simulink library "CommercialVehicleLibrary2G"  (R2021a)
settings: Solver=VariableStepAuto  StartTime=0.0  StopTime=10.0  RelTol=1e-3
values from neighbouring files (symbols this model uses):
  brake_input = [0   tmax ... (first row only)    [init_vehicle.m]    (also in run_Circle.m = [0  tmax; run_Coastdown.m = [0  2  tmax; run_DoubleLaneChangeDriver.m = [0   2  tmax; run_MaxAcc.m = [0  2  tmax)
  pose_t0 = [0 0 0 0]    [init_vehicle.m]    (also in run_Circle.m; run_Coastdown.m; run_DoubleLaneChangeDriver.m; run_MaxAcc.m)
  rdfname = 'TNO_FlatRoad.rdf'    [run_Circle.m]    (also in run_Coastdown.m; run_DoubleLaneChangeDriver.m; run_MaxAcc.m; run_Rollover.m)
  rdfname_inner = 'TNO_FlatRoad.rdf'    [run_Circle.m]    (also in run_Coastdown.m; run_DoubleLaneChangeDriver.m; run_MaxAcc.m; run_Rollover.m)
  steer_input = [0  tmax ... (first row only)    [init_vehicle.m]    (also in run_Circle.m = [0  2   10     13       tmax; run_Coastdown.m = [0 tmax; run_DoubleLaneChangeDriver.m = [0 tmax; run_MaxAcc.m = [0 tmax)
  throttle_input = [0         tmax ... (first row only)    [init_vehicle.m]    (also in run_Circle.m; run_Coastdown.m = [0        10         10.0001 tmax; run_DoubleLaneChangeDriver.m = [0        tmax; run_MaxAcc.m = [0        tmax)
  Vx = 0    [init_vehicle.m]    (also in run_Circle.m = Vx_kmh/3.6; run_Coastdown.m = Vx_kmh/3.6; run_DoubleLaneChangeDriver.m = Vx_kmh/3.6; run_MaxAcc.m)
  Vx_input = [0  tmax ... (first row only)    [init_vehicle.m]    (also in run_Circle.m; run_Coastdown.m = [0 tmax; run_DoubleLaneChangeDriver.m = [0 tmax; run_MaxAcc.m = [0 tmax)
undefined symbols (not defined in the file or in its folder): Drive, Floor, Fzstat, Fzstat1, Fzstat3, l, l_load1, l_load2, lbar, mass_load1, mass_load2, psi_semitrailer, rho, rim_Ixx, rim_Iyy, rim_mass, Steer, steer_path, tpfname, X, x_torsion, xcg, xcg1, xcg2, xcg_front, xcg_rear, xdrive1, xload1, xload2, xpos1, xref, xrev1, Xt0, Y, Yt0, Z
libraries: sm_lib x291, $bdroot x157, nesl_utility x143, vrlib x1
(part 5 of 12)

== system CommercialVehicleLibrary2G/Assemblies/Trailer load rear ==
  note: Measurements
  Bus Creator1 : BusCreator  Inputs=3
  Fcn1 : Fcn  Expr=u(2)
  Fcn2 : Fcn  Expr=u(2)
  "Load " : sm_lib/Body Elements/Brick Solid  GraphicAmbientColor=[0.15 0.15 0.15 1.0]  BasedOnType=Density  BrickDimensions=[l_load2 w h]  BrickDimensionUnits=m  CenterOfMass=[0 0 0]  CenterOfMassUnits=m  GraphicDiffuseColor=[1.0 1.0 0.2]  Density=1000  DensityUnits=kg/m^3  DoExposeReferenceFrame=on  GraphicEmissiveColor=[0.0 0.0 0.0 1.0]  ExportEntireGeometry=off  SerializedFrames=<Frames/>  MarkerShape=Sphere  MarkerSize=10  GraphicType=FromGeometry  InertiaType=Custom  Mass=mass_load  MassUnits=kg  MomentsOfInertia=[Ixx Iyy Izz]  MomentsOfInertiaUnits=kg*m^2  GraphicOpacity=0.5  ProductsOfInertia=[0 0 0]  ProductsOfInertiaUnits=kg*m^2  GraphicShininess=75  GraphicSpecularColor=[0.5 0.5 0.5 1.0]  GraphicVisPropType=SimpleVisualProperties
  Mux : Mux  Inputs=3
  Mux1 : Mux  Inputs=3
  Mux2 : Mux  Inputs=3
  PS-Simulink Converter : nesl_utility/PS-Simulink Converter  PhysicalDomain=network_engine_domain  SubClassName=ps_output  LeftPortType=input  RightPortType=output  PseudoPeriodic=off  Frequencies=[]  Unit=inherit  AffineConversion=off
      settings: SourceProductBaseCode=PW,SS
  PS-Simulink Converter{1..6} (6 alike) : nesl_utility/PS-Simulink Converter  PhysicalDomain=network_engine_domain  SubClassName=ps_output  LeftPortType=input  RightPortType=output  PseudoPeriodic=off  Frequencies=[]  Unit=m/s^2  AffineConversion=off
      settings: SourceProductBaseCode=PW,SS
  PS-Simulink Converter7 : nesl_utility/PS-Simulink Converter  PhysicalDomain=network_engine_domain  SubClassName=ps_output  LeftPortType=input  RightPortType=output  PseudoPeriodic=off  Frequencies=[]  Unit=inherit  AffineConversion=off
      settings: SourceProductBaseCode=PW,SS
  PS-Simulink Converter8 : nesl_utility/PS-Simulink Converter  PhysicalDomain=network_engine_domain  SubClassName=ps_output  LeftPortType=input  RightPortType=output  PseudoPeriodic=off  Frequencies=[]  Unit=inherit  AffineConversion=off
      settings: SourceProductBaseCode=PW,SS
  Transform Sensor : sm_lib/Frames and Transforms/Transform Sensor  MeasurementFrame=World  SenseAngle=off  SenseAxis=off  SenseAngle1=off  SenseAngle2=off  SenseAngle3=off  SenseQ=off  SenseR=off  SenseOmegaX=off  SenseOmegaY=off  SenseOmegaZ=off  SenseOmega1=off  SenseOmega2=off  SenseOmega3=off  SenseQDot=off  SenseRDot=off  SenseAlphaX=off  SenseAlphaY=off  SenseAlphaZ=off  SenseAlpha1=off  SenseAlpha2=off  SenseAlpha3=off  SenseQDDot=off  SenseRDDot=off  SenseX=on  SenseY=on  SenseZ=on  SenseRad=off  SenseAzim=off  SenseDist=off  SenseInc=off  SenseXDot=off  SenseYDot=off  SenseZDot=off  SenseRadDot=off  SenseAzimDot=off  SenseDistDot=off  SenseIncDot=off  SenseXDDot=off  SenseYDDot=off  SenseZDDot=off  SenseRadDDot=off  SenseAzimDDot=off  SenseDistDDot=off  SenseIncDDot=off
  Transform Sensor1 : sm_lib/Frames and Transforms/Transform Sensor  MeasurementFrame=NonRotatingFollower  SenseAngle=off  SenseAxis=off  SenseAngle1=off  SenseAngle2=off  SenseAngle3=off  SenseQ=off  SenseR=off  SenseOmegaX=off  SenseOmegaY=off  SenseOmegaZ=off  SenseOmega1=off  SenseOmega2=off  SenseOmega3=off  SenseQDot=off  SenseRDot=off  SenseAlphaX=off  SenseAlphaY=off  SenseAlphaZ=off  SenseAlpha1=off  SenseAlpha2=off  SenseAlpha3=off  SenseQDDot=off  SenseRDDot=off  SenseX=off  SenseY=off  SenseZ=off  SenseRad=off  SenseAzim=off  SenseDist=off  SenseInc=off  SenseXDot=off  SenseYDot=off  SenseZDot=off  SenseRadDot=off  SenseAzimDot=off  SenseDistDot=off  SenseIncDot=off  SenseXDDot=on  SenseYDDot=on  SenseZDDot=on  SenseRadDDot=off  SenseAzimDDot=off  SenseDistDDot=off  SenseIncDDot=off
  Transform Sensor2 : sm_lib/Frames and Transforms/Transform Sensor  MeasurementFrame=NonRotatingFollower  SenseAngle=off  SenseAxis=off  SenseAngle1=off  SenseAngle2=off  SenseAngle3=off  SenseQ=off  SenseR=off  SenseOmegaX=off  SenseOmegaY=off  SenseOmegaZ=off  SenseOmega1=off  SenseOmega2=off  SenseOmega3=off  SenseQDot=off  SenseRDot=off  SenseAlphaX=off  SenseAlphaY=off  SenseAlphaZ=off  SenseAlpha1=off  SenseAlpha2=off  SenseAlpha3=off  SenseQDDot=off  SenseRDDot=off  SenseX=off  SenseY=off  SenseZ=off  SenseRad=off  SenseAzim=off  SenseDist=off  SenseInc=off  SenseXDot=off  SenseYDot=off  SenseZDot=off  SenseRadDot=off  SenseAzimDot=off  SenseDistDot=off  SenseIncDot=off  SenseXDDot=on  SenseYDDot=on  SenseZDDot=on  SenseRadDDot=off  SenseAzimDDot=off  SenseDistDDot=off  SenseIncDDot=off
  Weld Joint : sm_lib/Joints/Weld Joint  JointMode=Normal  SenseConstraintForce=off  SenseConstraintForceX=off  SenseConstraintForceY=off  SenseConstraintForceZ=off  SenseConstraintTorque=off  SenseConstraintTorqueX=off  SenseConstraintTorqueY=off  SenseConstraintTorqueZ=off  SenseTotalForce=off  SenseTotalForceX=off  SenseTotalForceY=off  SenseTotalForceZ=off  SenseTotalTorque=off  SenseTotalTorqueX=off  SenseTotalTorqueY=off  SenseTotalTorqueZ=off  CompositeWrenchDir=FollowerOnBase  CompositeWrenchFrame=BaseFrame
  World Frame : sm_lib/Frames and Transforms/World Frame
  World Frame1 : sm_lib/Frames and Transforms/World Frame
  World Frame2 : sm_lib/Frames and Transforms/World Frame
  load_corner_pos : sm_lib/Frames and Transforms/Rigid Transform  TranslationMethod=Cartesian  TranslationStandardOffset=0  TranslationLengthUnit=m  TranslationStandardAxis=+Z  TranslationCartesianOffset=[(-0.5*l_load) 0 0]  TranslationROffset=0  TranslationROffsetUnits=m  TranslationZOffset=0  TranslationZOffsetUnits=m  TranslationThetaOffset=0  TranslationThetaOffsetUnits=deg  RotationMethod=None  RotationAngleUnits=deg  RotationStandardAxis=+Z  RotationAngle=0.0  RotationArbitraryAxis=[0 0 1]  FollAlignAxisA=+X  BaseAlignAxisA=+Y  FollAlignAxisB=+Y  BaseAlignAxisB=+Z  RotationSequenceAxes=FollowerAxes  RotationSequence=XYX  RotationSequenceAngles=[0 0 0]  RotationSequenceAnglesUnits=deg  RotationMatrix=[1 0 0; 0 1 0; 0 0 1]
  pos_load : sm_lib/Frames and Transforms/Rigid Transform  TranslationMethod=Cartesian  TranslationStandardOffset=0  TranslationLengthUnit=m  TranslationStandardAxis=+Z  TranslationCartesianOffset=[-xcg2+xload 0 zcg+0.1]  TranslationROffset=0  TranslationROffsetUnits=m  TranslationZOffset=0  TranslationZOffsetUnits=m  TranslationThetaOffset=0  TranslationThetaOffsetUnits=deg  RotationMethod=None  RotationAngleUnits=deg  RotationStandardAxis=+Z  RotationAngle=0.0  RotationArbitraryAxis=[0 0 1]  FollAlignAxisA=+X  BaseAlignAxisA=+Y  FollAlignAxisB=+Y  BaseAlignAxisB=+Z  RotationSequenceAxes=FollowerAxes  RotationSequence=XYX  RotationSequenceAngles=[0 0 0]  RotationSequenceAnglesUnits=deg  RotationMatrix=[1 0 0; 0 1 0; 0 0 1]
  Chassis : PMIOPort  Side=Left
  Out1 : Outport
  wires:
  PS-Simulink Converter7/1 -> Mux/2
  PS-Simulink Converter/1 -> Mux/1
  PS-Simulink Converter8/1 -> Mux/3
  PS-Simulink Converter3/1 -> Mux1/1
  Mux1/1 -> Fcn2/1
  Mux/1 -> [Load_pos]
  PS-Simulink Converter5/1 -> Mux1/3
  Fcn2/1 -> [Load_acc_center]
  PS-Simulink Converter4/1 -> Mux1/2
  [Load_acc_center] -> Bus Creator1/2  "acc_center"
  Bus Creator1/1 -> Out1/1
  [Load_pos] -> Bus Creator1/1  "pos"
  PS-Simulink Converter2/1 -> Mux2/2
  PS-Simulink Converter1/1 -> Mux2/1
  PS-Simulink Converter6/1 -> Mux2/3
  Mux2/1 -> Fcn1/1
  Fcn1/1 -> [Load_acc_corner]
  [Load_acc_corner] -> Bus Creator1/3  "acc_corner"
  connections:
  "Load "/RConn1 -- Transform Sensor2/RConn1 -- Transform Sensor/RConn1 -- load_corner_pos/LConn1 -- pos_load/RConn1
  PS-Simulink Converter8/LConn1 -- Transform Sensor/RConn4
  PS-Simulink Converter7/LConn1 -- Transform Sensor/RConn3
  PS-Simulink Converter4/LConn1 -- Transform Sensor2/RConn3
  World Frame/RConn1 -- Transform Sensor/LConn1
  PS-Simulink Converter3/LConn1 -- Transform Sensor2/RConn2
  PS-Simulink Converter5/LConn1 -- Transform Sensor2/RConn4
  PS-Simulink Converter/LConn1 -- Transform Sensor/RConn2
  World Frame2/RConn1 -- Transform Sensor2/LConn1
  pos_load/LConn1 -- Weld Joint/RConn1
  Weld Joint/LConn1 -- Chassis/RConn1
  PS-Simulink Converter6/LConn1 -- Transform Sensor1/RConn4
  World Frame1/RConn1 -- Transform Sensor1/LConn1
  Transform Sensor1/RConn1 -- load_corner_pos/RConn1
  PS-Simulink Converter1/LConn1 -- Transform Sensor1/RConn2
  PS-Simulink Converter2/LConn1 -- Transform Sensor1/RConn3

== system CommercialVehicleLibrary2G/Assemblies/Truck load ==
  note: Measurements
  Bus Creator1 : BusCreator  Inputs=3
  Fcn1 : Fcn  Expr=u(2)
  Fcn2 : Fcn  Expr=u(2)
  "Load " : sm_lib/Body Elements/Brick Solid  GraphicAmbientColor=[0.15 0.15 0.15 1.0]  BasedOnType=Density  BrickDimensions=[l_load w h]  BrickDimensionUnits=m  CenterOfMass=[0 0 0]  CenterOfMassUnits=m  GraphicDiffuseColor=[1.0 0.4 0.4]  Density=1000  DensityUnits=kg/m^3  DoExposeReferenceFrame=on  GraphicEmissiveColor=[0.0 0.0 0.0 1.0]  ExportEntireGeometry=off  SerializedFrames=<Frames/>  MarkerShape=Sphere  MarkerSize=10  GraphicType=FromGeometry  InertiaType=Custom  Mass=mass_load  MassUnits=kg  MomentsOfInertia=[Ixx Iyy Izz]  MomentsOfInertiaUnits=kg*m^2  GraphicOpacity=0.5  ProductsOfInertia=[0 0 0]  ProductsOfInertiaUnits=kg*m^2  GraphicShininess=75  GraphicSpecularColor=[0.5 0.5 0.5 1.0]  GraphicVisPropType=SimpleVisualProperties
  Mux : Mux  Inputs=3
  Mux1 : Mux  Inputs=3
  Mux2 : Mux  Inputs=3
  PS-Simulink Converter : nesl_utility/PS-Simulink Converter  PhysicalDomain=network_engine_domain  SubClassName=ps_output  LeftPortType=input  RightPortType=output  PseudoPeriodic=off  Frequencies=[]  Unit=inherit  AffineConversion=off
      settings: SourceProductBaseCode=PW,SS
  PS-Simulink Converter{1..6} (6 alike) : nesl_utility/PS-Simulink Converter  PhysicalDomain=network_engine_domain  SubClassName=ps_output  LeftPortType=input  RightPortType=output  PseudoPeriodic=off  Frequencies=[]  Unit=m/s^2  AffineConversion=off
      settings: SourceProductBaseCode=PW,SS
  PS-Simulink Converter7 : nesl_utility/PS-Simulink Converter  PhysicalDomain=network_engine_domain  SubClassName=ps_output  LeftPortType=input  RightPortType=output  PseudoPeriodic=off  Frequencies=[]  Unit=inherit  AffineConversion=off
      settings: SourceProductBaseCode=PW,SS
  PS-Simulink Converter8 : nesl_utility/PS-Simulink Converter  PhysicalDomain=network_engine_domain  SubClassName=ps_output  LeftPortType=input  RightPortType=output  PseudoPeriodic=off  Frequencies=[]  Unit=inherit  AffineConversion=off
      settings: SourceProductBaseCode=PW,SS
  Transform Sensor : sm_lib/Frames and Transforms/Transform Sensor  MeasurementFrame=World  SenseAngle=off  SenseAxis=off  SenseAngle1=off  SenseAngle2=off  SenseAngle3=off  SenseQ=off  SenseR=off  SenseOmegaX=off  SenseOmegaY=off  SenseOmegaZ=off  SenseOmega1=off  SenseOmega2=off  SenseOmega3=off  SenseQDot=off  SenseRDot=off  SenseAlphaX=off  SenseAlphaY=off  SenseAlphaZ=off  SenseAlpha1=off  SenseAlpha2=off  SenseAlpha3=off  SenseQDDot=off  SenseRDDot=off  SenseX=on  SenseY=on  SenseZ=on  SenseRad=off  SenseAzim=off  SenseDist=off  SenseInc=off  SenseXDot=off  SenseYDot=off  SenseZDot=off  SenseRadDot=off  SenseAzimDot=off  SenseDistDot=off  SenseIncDot=off  SenseXDDot=off  SenseYDDot=off  SenseZDDot=off  SenseRadDDot=off  SenseAzimDDot=off  SenseDistDDot=off  SenseIncDDot=off
  Transform Sensor1 : sm_lib/Frames and Transforms/Transform Sensor  MeasurementFrame=NonRotatingFollower  SenseAngle=off  SenseAxis=off  SenseAngle1=off  SenseAngle2=off  SenseAngle3=off  SenseQ=off  SenseR=off  SenseOmegaX=off  SenseOmegaY=off  SenseOmegaZ=off  SenseOmega1=off  SenseOmega2=off  SenseOmega3=off  SenseQDot=off  SenseRDot=off  SenseAlphaX=off  SenseAlphaY=off  SenseAlphaZ=off  SenseAlpha1=off  SenseAlpha2=off  SenseAlpha3=off  SenseQDDot=off  SenseRDDot=off  SenseX=off  SenseY=off  SenseZ=off  SenseRad=off  SenseAzim=off  SenseDist=off  SenseInc=off  SenseXDot=off  SenseYDot=off  SenseZDot=off  SenseRadDot=off  SenseAzimDot=off  SenseDistDot=off  SenseIncDot=off  SenseXDDot=on  SenseYDDot=on  SenseZDDot=on  SenseRadDDot=off  SenseAzimDDot=off  SenseDistDDot=off  SenseIncDDot=off
  Transform Sensor2 : sm_lib/Frames and Transforms/Transform Sensor  MeasurementFrame=NonRotatingFollower  SenseAngle=off  SenseAxis=off  SenseAngle1=off  SenseAngle2=off  SenseAngle3=off  SenseQ=off  SenseR=off  SenseOmegaX=off  SenseOmegaY=off  SenseOmegaZ=off  SenseOmega1=off  SenseOmega2=off  SenseOmega3=off  SenseQDot=off  SenseRDot=off  SenseAlphaX=off  SenseAlphaY=off  SenseAlphaZ=off  SenseAlpha1=off  SenseAlpha2=off  SenseAlpha3=off  SenseQDDot=off  SenseRDDot=off  SenseX=off  SenseY=off  SenseZ=off  SenseRad=off  SenseAzim=off  SenseDist=off  SenseInc=off  SenseXDot=off  SenseYDot=off  SenseZDot=off  SenseRadDot=off  SenseAzimDot=off  SenseDistDot=off  SenseIncDot=off  SenseXDDot=on  SenseYDDot=on  SenseZDDot=on  SenseRadDDot=off  SenseAzimDDot=off  SenseDistDDot=off  SenseIncDDot=off
  Weld Joint : sm_lib/Joints/Weld Joint  JointMode=Normal  SenseConstraintForce=off  SenseConstraintForceX=off  SenseConstraintForceY=off  SenseConstraintForceZ=off  SenseConstraintTorque=off  SenseConstraintTorqueX=off  SenseConstraintTorqueY=off  SenseConstraintTorqueZ=off  SenseTotalForce=off  SenseTotalForceX=off  SenseTotalForceY=off  SenseTotalForceZ=off  SenseTotalTorque=off  SenseTotalTorqueX=off  SenseTotalTorqueY=off  SenseTotalTorqueZ=off  CompositeWrenchDir=FollowerOnBase  CompositeWrenchFrame=BaseFrame
  World Frame : sm_lib/Frames and Transforms/World Frame
  World Frame1 : sm_lib/Frames and Transforms/World Frame
  World Frame2 : sm_lib/Frames and Transforms/World Frame
  load_corner_pos : sm_lib/Frames and Transforms/Rigid Transform  TranslationMethod=Cartesian  TranslationStandardOffset=0  TranslationLengthUnit=m  TranslationStandardAxis=+Z  TranslationCartesianOffset=[(-0.5*l_load) 0 0]  TranslationROffset=0  TranslationROffsetUnits=m  TranslationZOffset=0  TranslationZOffsetUnits=m  TranslationThetaOffset=0  TranslationThetaOffsetUnits=deg  RotationMethod=None  RotationAngleUnits=deg  RotationStandardAxis=+Z  RotationAngle=0.0  RotationArbitraryAxis=[0 0 1]  FollAlignAxisA=+X  BaseAlignAxisA=+Y  FollAlignAxisB=+Y  BaseAlignAxisB=+Z  RotationSequenceAxes=FollowerAxes  RotationSequence=XYX  RotationSequenceAngles=[0 0 0]  RotationSequenceAnglesUnits=deg  RotationMatrix=[1 0 0; 0 1 0; 0 0 1]
  pos_load : sm_lib/Frames and Transforms/Rigid Transform  TranslationMethod=Cartesian  TranslationStandardOffset=0  TranslationLengthUnit=m  TranslationStandardAxis=+Z  TranslationCartesianOffset=[-xcg_rear+xload 0 +zload+zcg-0.9]  TranslationROffset=0  TranslationROffsetUnits=m  TranslationZOffset=0  TranslationZOffsetUnits=m  TranslationThetaOffset=0  TranslationThetaOffsetUnits=deg  RotationMethod=None  RotationAngleUnits=deg  RotationStandardAxis=+Z  RotationAngle=0.0  RotationArbitraryAxis=[0 0 1]  FollAlignAxisA=+X  BaseAlignAxisA=+Y  FollAlignAxisB=+Y  BaseAlignAxisB=+Z  RotationSequenceAxes=FollowerAxes  RotationSequence=XYX  RotationSequenceAngles=[0 0 0]  RotationSequenceAnglesUnits=deg  RotationMatrix=[1 0 0; 0 1 0; 0 0 1]
  Chassis : PMIOPort  Side=Left
  Out1 : Outport
  wires:
  [Load_acc_corner] -> Bus Creator1/3  "acc_corner"
  Fcn1/1 -> [Load_acc_corner]
  Mux2/1 -> Fcn1/1
  PS-Simulink Converter6/1 -> Mux2/3
  PS-Simulink Converter1/1 -> Mux2/1
  PS-Simulink Converter2/1 -> Mux2/2
  [Load_pos] -> Bus Creator1/1  "pos"
  Bus Creator1/1 -> Out1/1
  [Load_acc_center] -> Bus Creator1/2  "acc_center"
  PS-Simulink Converter4/1 -> Mux1/2
  Fcn2/1 -> [Load_acc_center]
  PS-Simulink Converter5/1 -> Mux1/3
  Mux/1 -> [Load_pos]
  Mux1/1 -> Fcn2/1
  PS-Simulink Converter3/1 -> Mux1/1
  PS-Simulink Converter8/1 -> Mux/3
  PS-Simulink Converter/1 -> Mux/1
  PS-Simulink Converter7/1 -> Mux/2
  connections:
  PS-Simulink Converter2/LConn1 -- Transform Sensor1/RConn3
  PS-Simulink Converter1/LConn1 -- Transform Sensor1/RConn2
  Transform Sensor1/RConn1 -- load_corner_pos/RConn1
  World Frame1/RConn1 -- Transform Sensor1/LConn1
  PS-Simulink Converter6/LConn1 -- Transform Sensor1/RConn4
  Weld Joint/LConn1 -- Chassis/RConn1
  pos_load/LConn1 -- Weld Joint/RConn1
  World Frame2/RConn1 -- Transform Sensor2/LConn1
  PS-Simulink Converter/LConn1 -- Transform Sensor/RConn2
  PS-Simulink Converter5/LConn1 -- Transform Sensor2/RConn4
  PS-Simulink Converter3/LConn1 -- Transform Sensor2/RConn2
  World Frame/RConn1 -- Transform Sensor/LConn1
  PS-Simulink Converter4/LConn1 -- Transform Sensor2/RConn3
  PS-Simulink Converter7/LConn1 -- Transform Sensor/RConn3
  PS-Simulink Converter8/LConn1 -- Transform Sensor/RConn4
  pos_load/RConn1 -- load_corner_pos/LConn1 -- Transform Sensor/RConn1 -- Transform Sensor2/RConn1 -- "Load "/RConn1

== system CommercialVehicleLibrary2G/Combinations/LZV_A ==
  Bus Selector : BusSelector  OutputSignals=chassis.Vx,steeraxle.pos,driveaxle.pos
  Clock : Clock
  "Drawbar Trailer - 2 axle " : $bdroot/Trailers/Drawbar Trailer - 2 axle   xref=-15.06+1  l_chassis=7.82  lbar=2.0  mass_empty=3900  mass_load=13600  rho=350  Fzstat=8500*9.81
  Driver : $bdroot/Assemblies/Driver  SystemSampleTime=-1  VariantActivationTime=update diagram  Latency=0  AutoFrameSizeCalculation=off
  Semitrailer : $bdroot/Trailers/Semitrailer  xref=-3.06  xaxle2=8.475  lchassis=13.6  x5th=1.6  mass_empty=6000  mass_load=27000  rho=350  Fzstat=7200*9.81  lbdouble=0  psi_semitrailer=pose_t0(4)
  To Workspace : ToWorkspace  VariableName=p_time  SampleTime=-1
  To Workspace21 : ToWorkspace  VariableName=p_inputs_delta  SampleTime=-1
  To Workspace22 : ToWorkspace  VariableName=p_inputs_throttle  SampleTime=-1
  To Workspace23 : ToWorkspace  VariableName=p_inputs_brake  SampleTime=-1
  To_workspace_drawbar_trailer_2axle : $bdroot/Utilities/To_workspace_drawbar_trailer_2axle  SystemSampleTime=-1  VariantActivationTime=update diagram  Latency=0  AutoFrameSizeCalculation=off
  To_workspace_semitrailer : $bdroot/Utilities/To_workspace_semitrailer  SystemSampleTime=-1  VariantActivationTime=update diagram  Latency=0  AutoFrameSizeCalculation=off
  To_workspace_tractor : $bdroot/Utilities/To_workspace_tractor  SystemSampleTime=-1  VariantActivationTime=update diagram  Latency=0  AutoFrameSizeCalculation=off
  Tractor : $bdroot/Vehicles/Tractor  xref=0  xrear=-3.80  Fzstat1=7500*9.81  Fzstat2=11500*9.81  Xt0=pose_t0(1)  Yt0=pose_t0(2)  Psit0=pose_t0(3)
  wires:
  Driver/3 -> Tractor/3, To Workspace23/1
  Driver/2 -> Tractor/2, To Workspace22/1
  Clock/1 -> Driver/1, To Workspace/1
  Driver/1 -> Tractor/1, To Workspace21/1
  Tractor/1 -> To_workspace_tractor/1, Bus Selector/1
  Bus Selector/1 -> Driver/2  "<Vx>"
  Bus Selector/2 -> Driver/3  "<pos>"
  Bus Selector/3 -> Driver/4  "<pos>"
  Tractor/2 -> Semitrailer/1, "Drawbar Trailer - 2 axle "/1
  "Drawbar Trailer - 2 axle "/1 -> To_workspace_drawbar_trailer_2axle/1
  Semitrailer/1 -> To_workspace_semitrailer/1
  connections:
  Semitrailer/LConn1 -- Tractor/RConn1
  Semitrailer/RConn1 -- "Drawbar Trailer - 2 axle "/LConn1

== system CommercialVehicleLibrary2G/Combinations/LZV_B ==
  Bus Selector : BusSelector  OutputSignals=chassis.Vx,steeraxle.pos,driveaxle.pos
  Clock : Clock
  Driver : $bdroot/Assemblies/Driver  SystemSampleTime=-1  VariantActivationTime=update diagram  Latency=0  AutoFrameSizeCalculation=off
  Semitrailer : $bdroot/Trailers/Semitrailer  xref=-3.06  xaxle2=8.475  lchassis=12.0  x5th=1.6  mass_empty=5000  mass_load=14500  rho=350  Fzstat=6400*9.81  lbdouble=4.18  psi_semitrailer=pose_t0(4)
  Semitrailer1 : $bdroot/Trailers/Semitrailer  xref=-11.85  xaxle2=8.475  lchassis=13.6  x5th=1.6  mass_empty=6000  mass_load=25000  rho=350  Fzstat=6600*9.81  lbdouble=0  psi_semitrailer=pose_t0(4)
  To Workspace : ToWorkspace  VariableName=p_time  SampleTime=-1
  To Workspace21 : ToWorkspace  VariableName=p_inputs_delta  SampleTime=-1
  To Workspace22 : ToWorkspace  VariableName=p_inputs_throttle  SampleTime=-1
  To Workspace23 : ToWorkspace  VariableName=p_inputs_brake  SampleTime=-1
  To_workspace_semitrailer1 : Subsystem
  To_workspace_semitrailer2 : Subsystem
  To_workspace_tractor : $bdroot/Utilities/To_workspace_tractor  SystemSampleTime=-1  VariantActivationTime=update diagram  Latency=0  AutoFrameSizeCalculation=off
  Tractor : $bdroot/Vehicles/Tractor  xref=0  xrear=-3.80  Fzstat1=7500*9.81  Fzstat2=11500*9.81  Xt0=pose_t0(1)  Yt0=pose_t0(2)  Psit0=pose_t0(3)
  wires:
  Driver/3 -> Tractor/3, To Workspace23/1
  Driver/2 -> Tractor/2, To Workspace22/1
  Clock/1 -> Driver/1, To Workspace/1
  Driver/1 -> Tractor/1, To Workspace21/1
  Tractor/1 -> To_workspace_tractor/1, Bus Selector/1
  Bus Selector/1 -> Driver/2  "<Vx>"
  Bus Selector/2 -> Driver/3  "<pos>"
  Bus Selector/3 -> Driver/4  "<pos>"
  Semitrailer1/1 -> To_workspace_semitrailer2/1(In1)
  Tractor/2 -> Semitrailer1/1, Semitrailer/1
  Semitrailer/1 -> To_workspace_semitrailer1/1(In1)
  connections:
  Semitrailer/LConn1 -- Tractor/RConn1
  Semitrailer1/LConn1 -- Semitrailer/RConn1

== system CommercialVehicleLibrary2G/Combinations/LZV_C ==
  Bus Selector : BusSelector  OutputSignals=chassis.Vx,steeraxle1.pos,driveaxle2.pos
  Clock : Clock
  Driver : $bdroot/Assemblies/Driver  SystemSampleTime=-1  VariantActivationTime=update diagram  Latency=0  AutoFrameSizeCalculation=off
  Rigid Truck - 4 axles : $bdroot/Vehicles/Rigid Truck - 4 axles  xref=0  xaxle=5.1  l_chassis=12  l_load=9.6  mass_load=19000  rho=350  Fzstat1=7500*9.81  Fzstat2=7500*9.81  Fzstat3=8500*9.81  Fzstat4=8500*9.81  conf=Steer-Steer-Drive-Drive  Xt0=pose_t0(1)  Yt0=pose_t0(2)  Psit0=pose_t0(3)
  To Workspace : ToWorkspace  VariableName=p_time  SampleTime=-1
  To Workspace21 : ToWorkspace  VariableName=p_inputs_delta  SampleTime=-1
  To Workspace22 : ToWorkspace  VariableName=p_inputs_throttle  SampleTime=-1
  To Workspace23 : ToWorkspace  VariableName=p_inputs_brake  SampleTime=-1
  To_workspace_trailer_3axle : $bdroot/Utilities/To_workspace_trailer_3axle  SystemSampleTime=-1  VariantActivationTime=update diagram  Latency=0  AutoFrameSizeCalculation=off
  To_workspace_truck_4axle1 : $bdroot/Utilities/To_workspace_truck_4axle  SystemSampleTime=-1  VariantActivationTime=update diagram  Latency=0  AutoFrameSizeCalculation=off
  "Trailer - 3 axle " : $bdroot/Trailers/Trailer - 3 axle   xref=-10.0  xtrailer=5  l_chassis=10  lturn=1.2  lbar=2.7  mass_empty=6000  mass_load=22000  rho=350  Fzstat=9333*9.81
  wires:
  Driver/3 -> Rigid Truck - 4 axles/3, To Workspace23/1
  Driver/2 -> Rigid Truck - 4 axles/2, To Workspace22/1
  Clock/1 -> Driver/1, To Workspace/1
  Driver/1 -> Rigid Truck - 4 axles/1, To Workspace21/1
  Rigid Truck - 4 axles/1 -> To_workspace_truck_4axle1/1, Bus Selector/1
  Bus Selector/1 -> Driver/2  "<Vx>"
  Bus Selector/2 -> Driver/3  "<pos>"
  Bus Selector/3 -> Driver/4  "<pos>"
  "Trailer - 3 axle "/1 -> To_workspace_trailer_3axle/1
  Rigid Truck - 4 axles/2 -> "Trailer - 3 axle "/1
  connections:
  "Trailer - 3 axle "/LConn1 -- Rigid Truck - 4 axles/RConn1

== system CommercialVehicleLibrary2G/Combinations/LZV_D ==
  Bus Selector : BusSelector  OutputSignals=chassis.Vx,steeraxle.pos,driveaxle2.pos
  Clock : Clock
  Dolly : $bdroot/Trailers/Dolly  xref=-8.35  lbar=3.50  Fzstat=6700*9.81
  Driver : $bdroot/Assemblies/Driver  SystemSampleTime=-1  VariantActivationTime=update diagram  Latency=0  AutoFrameSizeCalculation=off
  Rigid Truck - 3 axles : $bdroot/Vehicles/Rigid Truck - 3 axles  xref=0  xaxle=5.0  l_load=7.82  mass_load=15000  rho=350  Fzstat1=7500*9.81  Fzstat2=9250*9.81  Fzstat3=9250*9.81  Xt0=pose_t0(1)  Yt0=pose_t0(2)  Psit0=pose_t0(3)
  Semitrailer : $bdroot/Trailers/Semitrailer  xref=-11.85  xaxle2=8.475  lchassis=13.6  x5th=1.6  mass_empty=6000  mass_load=26200  rho=350  Fzstat=6800*9.81  lbdouble=0  psi_semitrailer=pose_t0(4)
  To Workspace : ToWorkspace  VariableName=p_time  SampleTime=-1
  To Workspace21 : ToWorkspace  VariableName=p_inputs_delta  SampleTime=-1
  To Workspace22 : ToWorkspace  VariableName=p_inputs_throttle  SampleTime=-1
  To Workspace23 : ToWorkspace  VariableName=p_inputs_brake  SampleTime=-1
  To_workspace_dolly : $bdroot/Utilities/To_workspace_dolly  SystemSampleTime=-1  VariantActivationTime=update diagram  Latency=0  AutoFrameSizeCalculation=off
  To_workspace_semitrailer : $bdroot/Utilities/To_workspace_semitrailer  SystemSampleTime=-1  VariantActivationTime=update diagram  Latency=0  AutoFrameSizeCalculation=off
  To_workspace_truck_3axle : $bdroot/Utilities/To_workspace_truck_3axle  SystemSampleTime=-1  VariantActivationTime=update diagram  Latency=0  AutoFrameSizeCalculation=off
  wires:
  Driver/3 -> Rigid Truck - 3 axles/3, To Workspace23/1
  Driver/2 -> Rigid Truck - 3 axles/2, To Workspace22/1
  Clock/1 -> Driver/1, To Workspace/1
  Driver/1 -> Rigid Truck - 3 axles/1, To Workspace21/1
  Rigid Truck - 3 axles/1 -> To_workspace_truck_3axle/1, Bus Selector/1
  Bus Selector/1 -> Driver/2  "<Vx>"
  Dolly/1 -> To_workspace_dolly/1
  Bus Selector/2 -> Driver/3  "<pos>"
  Bus Selector/3 -> Driver/4  "<pos>"
  Rigid Truck - 3 axles/2 -> Semitrailer/1, Dolly/1
  Semitrailer/1 -> To_workspace_semitrailer/1
  connections:
  Dolly/LConn1 -- Rigid Truck - 3 axles/RConn1
  Semitrailer/LConn1 -- Dolly/RConn1

== system CommercialVehicleLibrary2G/Combinations/LZV_E ==
  Bus Selector : BusSelector  OutputSignals=chassis.Vx,steeraxle.pos,driveaxle2.pos
  Clock : Clock
  "Drawbar Trailer - 2 axle 1 " : $bdroot/Trailers/Drawbar Trailer - 2 axle   xref=-7.82  l_chassis=6.5  lbar=2.0  mass_empty=4000  mass_load=13000  rho=350  Fzstat=8600*9.81
  Drawbar Trailer - 2 axle 2 : $bdroot/Trailers/Drawbar Trailer - 2 axle   xref=-15.32  l_chassis=6.5  lbar=2.0  mass_empty=4000  mass_load=13000  rho=350  Fzstat=8250*9.81
  Driver : $bdroot/Assemblies/Driver  SystemSampleTime=-1  VariantActivationTime=update diagram  Latency=0  AutoFrameSizeCalculation=off
  Rigid Truck - 3 axles : $bdroot/Vehicles/Rigid Truck - 3 axles  xref=0  xaxle=5.0  l_load=7.82  mass_load=15000  rho=350  Fzstat1=7400*9.81  Fzstat2=9450*9.81  Fzstat3=9450*9.81  Xt0=pose_t0(1)  Yt0=pose_t0(2)  Psit0=pose_t0(3)
  To Workspace : ToWorkspace  VariableName=p_time  SampleTime=-1
  To Workspace21 : ToWorkspace  VariableName=p_inputs_delta  SampleTime=-1
  To Workspace22 : ToWorkspace  VariableName=p_inputs_throttle  SampleTime=-1
  To Workspace23 : ToWorkspace  VariableName=p_inputs_brake  SampleTime=-1
  To_workspace_drawbar_trailer_2axle : $bdroot/Utilities/To_workspace_drawbar_trailer_2axle  SystemSampleTime=-1  VariantActivationTime=update diagram  Latency=0  AutoFrameSizeCalculation=off
  To_workspace_drawbar_trailer_2axle 2 : Subsystem
  To_workspace_truck_3axle : $bdroot/Utilities/To_workspace_truck_3axle  SystemSampleTime=-1  VariantActivationTime=update diagram  Latency=0  AutoFrameSizeCalculation=off
  wires:
  Driver/3 -> Rigid Truck - 3 axles/3, To Workspace23/1
  Driver/2 -> Rigid Truck - 3 axles/2, To Workspace22/1
  Clock/1 -> Driver/1, To Workspace/1
  Driver/1 -> Rigid Truck - 3 axles/1, To Workspace21/1
  Rigid Truck - 3 axles/1 -> To_workspace_truck_3axle/1, Bus Selector/1
  Bus Selector/1 -> Driver/2  "<Vx>"
  "Drawbar Trailer - 2 axle 1 "/1 -> To_workspace_drawbar_trailer_2axle/1
  Bus Selector/2 -> Driver/3  "<pos>"
  Bus Selector/3 -> Driver/4  "<pos>"
  Rigid Truck - 3 axles/2 -> Drawbar Trailer - 2 axle 2/1, "Drawbar Trailer - 2 axle 1 "/1
  Drawbar Trailer - 2 axle 2/1 -> To_workspace_drawbar_trailer_2axle 2/1(In1)
  connections:
  "Drawbar Trailer - 2 axle 1 "/LConn1 -- Rigid Truck - 3 axles/RConn1
  Drawbar Trailer - 2 axle 2/LConn1 -- "Drawbar Trailer - 2 axle 1 "/RConn1

== system CommercialVehicleLibrary2G/Combinations/LZV_F ==
  Bus Selector : BusSelector  OutputSignals=chassis.Vx,steeraxle1.pos,driveaxle2.pos
  Clock : Clock
  Driver : $bdroot/Assemblies/Driver  SystemSampleTime=-1  VariantActivationTime=update diagram  Latency=0  AutoFrameSizeCalculation=off
  Rigid Truck - 4 axles : $bdroot/Vehicles/Rigid Truck - 4 axles  xref=0  xaxle=5.25  l_chassis=10.1  l_load=5  mass_load=10000  rho=350  Fzstat1=7500*9.81  Fzstat2=7500*9.81  Fzstat3=10000*9.81  Fzstat4=10000*9.81  conf=Steer-Drive-Drive-Steer  Xt0=pose_t0(1)  Yt0=pose_t0(2)  Psit0=pose_t0(3)
  Semitrailer : $bdroot/Trailers/Semitrailer  xref=-8.4  xaxle2=8.475  lchassis=13.6  x5th=1.6  mass_empty=6000  mass_load=27000  rho=350  Fzstat=7000*9.81  lbdouble=0  psi_semitrailer=pose_t0(4)
  To Workspace : ToWorkspace  VariableName=p_time  SampleTime=-1
  To Workspace21 : ToWorkspace  VariableName=p_inputs_delta  SampleTime=-1
  To Workspace22 : ToWorkspace  VariableName=p_inputs_throttle  SampleTime=-1
  To Workspace23 : ToWorkspace  VariableName=p_inputs_brake  SampleTime=-1
  To_workspace_semitrailer : $bdroot/Utilities/To_workspace_semitrailer  SystemSampleTime=-1  VariantActivationTime=update diagram  Latency=0  AutoFrameSizeCalculation=off
  To_workspace_truck_4axle : $bdroot/Utilities/To_workspace_truck_4axle  SystemSampleTime=-1  VariantActivationTime=update diagram  Latency=0  AutoFrameSizeCalculation=off
  wires:
  Driver/3 -> Rigid Truck - 4 axles/3, To Workspace23/1
  Driver/2 -> Rigid Truck - 4 axles/2, To Workspace22/1
  Clock/1 -> Driver/1, To Workspace/1
  Driver/1 -> Rigid Truck - 4 axles/1, To Workspace21/1
  Rigid Truck - 4 axles/1 -> To_workspace_truck_4axle/1, Bus Selector/1
  Bus Selector/1 -> Driver/2  "<Vx>"
  Bus Selector/2 -> Driver/3  "<pos>"
  Bus Selector/3 -> Driver/4  "<pos>"
  Rigid Truck - 4 axles/2 -> Semitrailer/1
  Semitrailer/1 -> To_workspace_semitrailer/1
  connections:
  Semitrailer/LConn1 -- Rigid Truck - 4 axles/RConn1

== system CommercialVehicleLibrary2G/Combinations/LZV_G ==
  Bus Selector : BusSelector  OutputSignals=chassis.Vx,steeraxle1.pos,driveaxle2.pos
  Clock : Clock
  "Drawbar Trailer - 3 axle " : $bdroot/Trailers/Drawbar Trailer - 3 axle   xref=-9.6  l_chassis=10.0  lbar=2.0  mass_empty=6000  mass_load=22000  rho=350  Fzstat=9100*9.81
  Driver : $bdroot/Assemblies/Driver  SystemSampleTime=-1  VariantActivationTime=update diagram  Latency=0  AutoFrameSizeCalculation=off
  Rigid Truck - 4 axles : $bdroot/Vehicles/Rigid Truck - 4 axles  xref=0  xaxle=5.1  l_chassis=12  l_load=9.6  mass_load=19000  rho=350  Fzstat1=7400*9.81  Fzstat2=7400*9.81  Fzstat3=8900*9.81  Fzstat4=8900*9.81  conf=Steer-Steer-Drive-Drive  Xt0=pose_t0(1)  Yt0=pose_t0(2)  Psit0=pose_t0(3)
  To Workspace : ToWorkspace  VariableName=p_time  SampleTime=-1
  To Workspace21 : ToWorkspace  VariableName=p_inputs_delta  SampleTime=-1
  To Workspace22 : ToWorkspace  VariableName=p_inputs_throttle  SampleTime=-1
  To Workspace23 : ToWorkspace  VariableName=p_inputs_brake  SampleTime=-1
  To_workspace_drawbar_trailer_3axle : $bdroot/Utilities/To_workspace_drawbar_trailer_3axle  SystemSampleTime=-1  VariantActivationTime=update diagram  Latency=0  AutoFrameSizeCalculation=off
  To_workspace_truck_4axle : $bdroot/Utilities/To_workspace_truck_4axle  SystemSampleTime=-1  VariantActivationTime=update diagram  Latency=0  AutoFrameSizeCalculation=off
  wires:
  Driver/3 -> Rigid Truck - 4 axles/3, To Workspace23/1
  Driver/2 -> Rigid Truck - 4 axles/2, To Workspace22/1
  Clock/1 -> Driver/1, To Workspace/1
  Driver/1 -> Rigid Truck - 4 axles/1, To Workspace21/1
  Rigid Truck - 4 axles/1 -> To_workspace_truck_4axle/1, Bus Selector/1
  Bus Selector/1 -> Driver/2  "<Vx>"
  Bus Selector/2 -> Driver/3  "<pos>"
  Bus Selector/3 -> Driver/4  "<pos>"
  Rigid Truck - 4 axles/2 -> "Drawbar Trailer - 3 axle "/1
  "Drawbar Trailer - 3 axle "/1 -> To_workspace_drawbar_trailer_3axle/1
  connections:
  "Drawbar Trailer - 3 axle "/LConn1 -- Rigid Truck - 4 axles/RConn1

== system CommercialVehicleLibrary2G/Combinations/Tractor_semitrailer  ==
  Bus Selector : BusSelector  OutputSignals=chassis.Vx,steeraxle.Steeraxle_pos,driveaxle.Driveaxle_pos
  Clock : Clock
  Driver : $bdroot/Assemblies/Driver  SystemSampleTime=-1  VariantActivationTime=update diagram  Latency=0  AutoFrameSizeCalculation=off
  Semitrailer : $bdroot/Trailers/Semitrailer  xref=-3.06  xaxle2=8.475  lchassis=13.6  x5th=1.6  mass_empty=6000  mass_load=27000  rho=350  Fzstat=7000*9.81  lbdouble=0  psi_semitrailer=pose_t0(4)
  To Workspace : ToWorkspace  VariableName=p_time  SampleTime=-1
  To Workspace21 : ToWorkspace  VariableName=p_inputs_delta  SampleTime=-1
  To Workspace22 : ToWorkspace  VariableName=p_inputs_throttle  SampleTime=-1
  To Workspace23 : ToWorkspace  VariableName=p_inputs_brake  SampleTime=-1
  To_workspace_semitrailer : $bdroot/Utilities/To_workspace_semitrailer  SystemSampleTime=-1  VariantActivationTime=update diagram  Latency=0  AutoFrameSizeCalculation=off
  To_workspace_tractor : $bdroot/Utilities/To_workspace_tractor  SystemSampleTime=-1  VariantActivationTime=update diagram  Latency=0  AutoFrameSizeCalculation=off
  Tractor : $bdroot/Vehicles/Tractor  xref=0  xrear=-3.80  Fzstat1=7500*9.81  Fzstat2=11500*9.81  Xt0=pose_t0(1)  Yt0=pose_t0(2)  Psit0=pose_t0(3)
  wires:
  Driver/3 -> Tractor/3, To Workspace23/1
  Driver/2 -> Tractor/2, To Workspace22/1
  Clock/1 -> Driver/1, To Workspace/1
  Driver/1 -> Tractor/1, To Workspace21/1
  Tractor/1 -> To_workspace_tractor/1, Bus Selector/1
  Semitrailer/1 -> To_workspace_semitrailer/1
  Bus Selector/1 -> Driver/2  "<Vx>"
  Tractor/2 -> Semitrailer/1
  Bus Selector/2 -> Driver/3  "<Steeraxle_pos>"
  Bus Selector/3 -> Driver/4  "<Driveaxle_pos>"
  connections:
  Semitrailer/LConn1 -- Tractor/RConn1

== system CommercialVehicleLibrary2G/Combinations/Truck_dbtrailer ==
  Bus Selector : BusSelector  OutputSignals=chassis.Vx,steeraxle.pos,driveaxle2.pos
  Clock : Clock
  "Drawbar Trailer - 2 axle " : $bdroot/Trailers/Drawbar Trailer - 2 axle   xref=-7.82  l_chassis=7.5  lbar=2.0  mass_empty=4000  mass_load=10000  rho=250  Fzstat=6800*9.81
  Driver : $bdroot/Assemblies/Driver  SystemSampleTime=-1  VariantActivationTime=update diagram  Latency=0  AutoFrameSizeCalculation=off
  Rigid Truck - 3 axles : $bdroot/Vehicles/Rigid Truck - 3 axles  xref=0  xaxle=5.0  l_load=7.82  mass_load=15000  rho=350  Fzstat1=7400*9.81  Fzstat2=9450*9.81  Fzstat3=9450*9.81  Xt0=pose_t0(1)  Yt0=pose_t0(2)  Psit0=pose_t0(3)
  To Workspace : ToWorkspace  VariableName=p_time  SampleTime=-1
  To Workspace21 : ToWorkspace  VariableName=p_inputs_delta  SampleTime=-1
  To Workspace22 : ToWorkspace  VariableName=p_inputs_throttle  SampleTime=-1
  To Workspace23 : ToWorkspace  VariableName=p_inputs_brake  SampleTime=-1
  To_workspace_drawbar_trailer_2axle : $bdroot/Utilities/To_workspace_drawbar_trailer_2axle  SystemSampleTime=-1  VariantActivationTime=update diagram  Latency=0  AutoFrameSizeCalculation=off
  To_workspace_truck_3axle : $bdroot/Utilities/To_workspace_truck_3axle  SystemSampleTime=-1  VariantActivationTime=update diagram  Latency=0  AutoFrameSizeCalculation=off
  wires:
  Driver/3 -> Rigid Truck - 3 axles/3, To Workspace23/1
  Driver/2 -> Rigid Truck - 3 axles/2, To Workspace22/1
  Clock/1 -> Driver/1, To Workspace/1
  Driver/1 -> To Workspace21/1, Rigid Truck - 3 axles/1
  Rigid Truck - 3 axles/1 -> To_workspace_truck_3axle/1, Bus Selector/1
  Bus Selector/1 -> Driver/2  "<Vx>"
  "Drawbar Trailer - 2 axle "/1 -> To_workspace_drawbar_trailer_2axle/1
  Bus Selector/2 -> Driver/3  "<pos>"
  Bus Selector/3 -> Driver/4  "<pos>"
  Rigid Truck - 3 axles/2 -> "Drawbar Trailer - 2 axle "/1
  connections:
  "Drawbar Trailer - 2 axle "/LConn1 -- Rigid Truck - 3 axles/RConn1

== system CommercialVehicleLibrary2G/Combinations/Truck_trailer ==
  Bus Selector : BusSelector  OutputSignals=chassis.Vx,driveaxle.pos,steeraxle.pos
  Clock : Clock
  Driver : $bdroot/Assemblies/Driver  SystemSampleTime=-1  VariantActivationTime=update diagram  Latency=0  AutoFrameSizeCalculation=off
  Rigid Truck - 2 axles : $bdroot/Vehicles/Rigid Truck - 2 axles  xref=0  xaxle=5.9  l_load=7.5  mass_load=10000  rho=250  Fzstat1=7500*9.81  Fzstat2=11500*9.81  Xt0=pose_t0(1)  Yt0=pose_t0(2)  Psit0=pose_t0(3)
  To Workspace : ToWorkspace  VariableName=p_time  SampleTime=-1
  To Workspace21 : ToWorkspace  VariableName=p_inputs_delta  SampleTime=-1
  To Workspace22 : ToWorkspace  VariableName=p_inputs_throttle  SampleTime=-1
  To Workspace23 : ToWorkspace  VariableName=p_inputs_brake  SampleTime=-1
  To_workspace_trailer_2axle : $bdroot/Utilities/To_workspace_trailer_2axle  SystemSampleTime=-1  VariantActivationTime=update diagram  Latency=0  AutoFrameSizeCalculation=off
  To_workspace_truck_2axle : $bdroot/Utilities/To_workspace_truck_2axle  SystemSampleTime=-1  VariantActivationTime=update diagram  Latency=0  AutoFrameSizeCalculation=off
  "Trailer - 2 axle " : $bdroot/Trailers/Trailer - 2 axle   xref=-8.03  xtrailer=5.42  l_chassis=7.82  lturn=1.2  lbar=2.7  mass_empty=5000  mass_load=10000  rho=250  Fzstat=7500*9.81
  wires:
  Driver/3 -> Rigid Truck - 2 axles/3, To Workspace23/1
  Driver/2 -> Rigid Truck - 2 axles/2, To Workspace22/1
  Clock/1 -> Driver/1, To Workspace/1
  Driver/1 -> Rigid Truck - 2 axles/1, To Workspace21/1
  Rigid Truck - 2 axles/1 -> To_workspace_truck_2axle/1, Bus Selector/1
  Bus Selector/1 -> Driver/2  "<Vx>"
  Bus Selector/2 -> Driver/3  "<pos>"
  Bus Selector/3 -> Driver/4  "<pos>"
  "Trailer - 2 axle "/1 -> To_workspace_trailer_2axle/1
  Rigid Truck - 2 axles/2 -> "Trailer - 2 axle "/1
  connections:
  "Trailer - 2 axle "/LConn1 -- Rigid Truck - 2 axles/RConn1

== system CommercialVehicleLibrary2G/Components/5th Wheel Joint ==
  5th wheel joint : sm_lib/Joints/Revolute Joint  JointMode=Normal  SenseConstraintForce=off  SenseConstraintForceX=off  SenseConstraintForceY=off  SenseConstraintForceZ=off  SenseConstraintTorque=off  SenseConstraintTorqueX=off  SenseConstraintTorqueY=off  SenseConstraintTorqueZ=off  SenseTotalForce=off  SenseTotalForceX=off  SenseTotalForceY=off  SenseTotalForceZ=off  SenseTotalTorque=off  SenseTotalTorqueX=off  SenseTotalTorqueY=off  SenseTotalTorqueZ=off  CompositeWrenchDir=FollowerOnBase  CompositeWrenchFrame=BaseFrame  EquilibriumPosition=0  EquilibriumPositionUnits=deg  SpringStiffness=0  SpringStiffnessUnits=N*m/deg  DampingCoefficient=0  DampingCoefficientUnits=N*m/(deg/s)  TorqueActuationMode=NoTorque  MotionActuationMode=ComputedMotion  SensePosition=off  SenseVelocity=off  SenseAcceleration=off  SenseTorqueForce=off  SenseLowerLimitTorqueForce=off  SenseUpperLimitTorqueForce=off  LowerLimitSpecify=off  LowerLimitBound=-90  LowerLimitBoundUnits=deg  LowerLimitStiffness=1e4  LowerLimitStiffnessUnits=N*m/deg  LowerLimitDamping=10  LowerLimitDampingUnits=N*m/(deg/s)  LowerLimitTransitionRegionWidth=0.1  LowerLimitTransitionRegionWidthUnits=deg  UpperLimitSpecify=off  UpperLimitBound=90  UpperLimitBoundUnits=deg  UpperLimitStiffness=1e4  UpperLimitStiffnessUnits=N*m/deg  UpperLimitDamping=10  UpperLimitDampingUnits=N*m/(deg/s)  UpperLimitTransitionRegionWidth=0.1  UpperLimitTransitionRegionWidthUnits=deg  PositionTargetSpecify=on  PositionTargetPriority=High  PositionTargetValue=-psi_semitrailer  PositionTargetValueUnits=rad  VelocityTargetSpecify=off  VelocityTargetPriority=High  VelocityTargetValue=0  VelocityTargetValueUnits=deg/s
  5th wheel joint - axis : sm_lib/Joints/Revolute Joint  JointMode=Normal  SenseConstraintForce=off  SenseConstraintForceX=off  SenseConstraintForceY=off  SenseConstraintForceZ=off  SenseConstraintTorque=off  SenseConstraintTorqueX=off  SenseConstraintTorqueY=off  SenseConstraintTorqueZ=off  SenseTotalForce=off  SenseTotalForceX=off  SenseTotalForceY=off  SenseTotalForceZ=off  SenseTotalTorque=off  SenseTotalTorqueX=off  SenseTotalTorqueY=off  SenseTotalTorqueZ=off  CompositeWrenchDir=FollowerOnBase  CompositeWrenchFrame=BaseFrame  EquilibriumPosition=0  EquilibriumPositionUnits=deg  SpringStiffness=0  SpringStiffnessUnits=N*m/deg  DampingCoefficient=0  DampingCoefficientUnits=N*m/(deg/s)  TorqueActuationMode=NoTorque  MotionActuationMode=ComputedMotion  SensePosition=off  SenseVelocity=off  SenseAcceleration=off  SenseTorqueForce=off  SenseLowerLimitTorqueForce=off  SenseUpperLimitTorqueForce=off  LowerLimitSpecify=off  LowerLimitBound=-90  LowerLimitBoundUnits=deg  LowerLimitStiffness=1e4  LowerLimitStiffnessUnits=N*m/deg  LowerLimitDamping=10  LowerLimitDampingUnits=N*m/(deg/s)  LowerLimitTransitionRegionWidth=0.1  LowerLimitTransitionRegionWidthUnits=deg  UpperLimitSpecify=off  UpperLimitBound=90  UpperLimitBoundUnits=deg  UpperLimitStiffness=1e4  UpperLimitStiffnessUnits=N*m/deg  UpperLimitDamping=10  UpperLimitDampingUnits=N*m/(deg/s)  UpperLimitTransitionRegionWidth=0.1  UpperLimitTransitionRegionWidthUnits=deg  PositionTargetSpecify=off  PositionTargetPriority=High  PositionTargetValue=0  PositionTargetValueUnits=deg  VelocityTargetSpecify=off  VelocityTargetPriority=High  VelocityTargetValue=0  VelocityTargetValueUnits=deg/s
  Align_5th wheel : sm_lib/Frames and Transforms/Rigid Transform  TranslationMethod=None  TranslationStandardOffset=0  TranslationLengthUnit=m  TranslationStandardAxis=+Z  TranslationCartesianOffset=[0 0 0]  TranslationROffset=0  TranslationROffsetUnits=m  TranslationZOffset=0  TranslationZOffsetUnits=m  TranslationThetaOffset=0  TranslationThetaOffsetUnits=deg  RotationMethod=AlignedAxes  RotationAngleUnits=deg  RotationStandardAxis=+Z  RotationAngle=0.0  RotationArbitraryAxis=[0 0 1]  FollAlignAxisA=+Z  BaseAlignAxisA=+Y  FollAlignAxisB=+X  BaseAlignAxisB=+X  RotationSequenceAxes=FollowerAxes  RotationSequence=XYX  RotationSequenceAngles=[0 0 0]  RotationSequenceAnglesUnits=deg  RotationMatrix=[1 0 0; 0 1 0; 0 0 1]
  Realign_5th wheel : sm_lib/Frames and Transforms/Rigid Transform  TranslationMethod=None  TranslationStandardOffset=0  TranslationLengthUnit=m  TranslationStandardAxis=+Z  TranslationCartesianOffset=[0 0 0]  TranslationROffset=0  TranslationROffsetUnits=m  TranslationZOffset=0  TranslationZOffsetUnits=m  TranslationThetaOffset=0  TranslationThetaOffsetUnits=deg  RotationMethod=AlignedAxes  RotationAngleUnits=deg  RotationStandardAxis=+Z  RotationAngle=0.0  RotationArbitraryAxis=[0 0 1]  FollAlignAxisA=+Y  BaseAlignAxisA=+Z  FollAlignAxisB=+X  BaseAlignAxisB=+X  RotationSequenceAxes=FollowerAxes  RotationSequence=XYX  RotationSequenceAngles=[0 0 0]  RotationSequenceAnglesUnits=deg  RotationMatrix=[1 0 0; 0 1 0; 0 0 1]
  pos_5th Wheel : sm_lib/Frames and Transforms/Rigid Transform  TranslationMethod=Cartesian  TranslationStandardOffset=0  TranslationLengthUnit=m  TranslationStandardAxis=+Z  TranslationCartesianOffset=[xref 0 1.15]  TranslationROffset=0  TranslationROffsetUnits=m  TranslationZOffset=0  TranslationZOffsetUnits=m  TranslationThetaOffset=0  TranslationThetaOffsetUnits=deg  RotationMethod=None  RotationAngleUnits=deg  RotationStandardAxis=+Z  RotationAngle=0.0  RotationArbitraryAxis=[0 0 1]  FollAlignAxisA=+X  BaseAlignAxisA=+Y  FollAlignAxisB=+Y  BaseAlignAxisB=+Z  RotationSequenceAxes=FollowerAxes  RotationSequence=XYX  RotationSequenceAngles=[0 0 0]  RotationSequenceAnglesUnits=deg  RotationMatrix=[1 0 0; 0 1 0; 0 0 1]
  pos_trailer_front : sm_lib/Frames and Transforms/Rigid Transform  TranslationMethod=Cartesian  TranslationStandardOffset=1.8  TranslationLengthUnit=m  TranslationStandardAxis=-X  TranslationCartesianOffset=[-xref+xcg1 0 0.05]  TranslationROffset=0  TranslationROffsetUnits=m  TranslationZOffset=0  TranslationZOffsetUnits=m  TranslationThetaOffset=0  TranslationThetaOffsetUnits=deg  RotationMethod=None  RotationAngleUnits=deg  RotationStandardAxis=+Z  RotationAngle=0.0  RotationArbitraryAxis=[0 0 1]  FollAlignAxisA=+X  BaseAlignAxisA=+Y  FollAlignAxisB=+Y  BaseAlignAxisB=+Z  RotationSequenceAxes=FollowerAxes  RotationSequence=XYX  RotationSequenceAngles=[0 0 0]  RotationSequenceAnglesUnits=deg  RotationMatrix=[1 0 0; 0 1 0; 0 0 1]
  Chassis : PMIOPort  Side=Left
  Trailer : PMIOPort  Port=2  Side=Right
  connections:
  Align_5th wheel/RConn1 -- 5th wheel joint - axis/LConn1
  5th wheel joint - axis/RConn1 -- Realign_5th wheel/LConn1
  5th wheel joint/LConn1 -- Realign_5th wheel/RConn1
  5th wheel joint/RConn1 -- pos_trailer_front/LConn1
  pos_trailer_front/RConn1 -- Trailer/RConn1
  Align_5th wheel/LConn1 -- pos_5th Wheel/RConn1
  pos_5th Wheel/LConn1 -- Chassis/RConn1

== system CommercialVehicleLibrary2G/Components/Brake//Wheel_bearing ==
  Mdrive : Inport
  Mbrake : Inport  Port=2
  Look-Up Table : Lookup  InputValues=[-5:0.05:5]  Table=-tanh(2*[-5:0.05:5])  SaturateOnIntegerOverflow=on
  Product1 : Product  InputSameDT=on  SaturateOnIntegerOverflow=on  OutDataTypeStr=Inherit: Same as first input
  Rotational joint around y axis : Subsystem
  Sum : Sum  Inputs=++|
  axle : PMIOPort  Side=Left
  wheel : PMIOPort  Port=2  Side=Right
  omega : Outport  VectorParamsAs1DForOutWhenUnconnected=off
  wires:
  Sum/1 -> Rotational joint around y axis/1(Torque)
  Rotational joint around y axis/1(Rotational speed) -> Look-Up Table/1, omega/1
  Mdrive/1 -> Sum/1
  Product1/1 -> Sum/2
  Look-Up Table/1 -> Product1/2
  Mbrake/1 -> Product1/1
  connections:
  wheel/RConn1 -- Rotational joint around y axis/RConn1
  Rotational joint around y axis/LConn1 -- axle/RConn1

== system CommercialVehicleLibrary2G/Components/Braking system ==
  input (0-1) : Inport
  Mux : Mux  Inputs=2
  Mux1 : Mux  Inputs=2
  Mux2 : Mux  Inputs=2
  Saturation : Saturate  UpperLimit=1  LowerLimit=0
  brake moment gain1 : Gain  Gain=20000  SaturateOnIntegerOverflow=on  OutDataTypeStr=Inherit: Same as input  ParamDataTypeStr=Inherit: Same as input
  brake moment gain2 : Gain  Gain=28000  SaturateOnIntegerOverflow=on  OutDataTypeStr=Inherit: Same as input  ParamDataTypeStr=Inherit: Same as input
  brake moment gain3 : Gain  Gain=15000  SaturateOnIntegerOverflow=on  OutDataTypeStr=Inherit: Same as input  ParamDataTypeStr=Inherit: Same as input
  Mb_rear : Outport  VectorParamsAs1DForOutWhenUnconnected=off
  Mb_front : Outport  Port=2  VectorParamsAs1DForOutWhenUnconnected=off
  Mb_trailer : Outport  Port=3  VectorParamsAs1DForOutWhenUnconnected=off
  wires:
  Saturation/1 -> brake moment gain3/1, brake moment gain2/1, brake moment gain1/1
  Mux1/1 -> Mb_rear/1
  Mux2/1 -> Mb_front/1
  brake moment gain3/1 -> Mux/2, Mux/1
  input (0-1)/1 -> Saturation/1
  Mux/1 -> Mb_trailer/1
  brake moment gain2/1 -> Mux1/2, Mux1/1
  brake moment gain1/1 -> Mux2/2, Mux2/1
